simulink model "subsampling"  (R2025b)
settings: Solver=FixedStepAuto  StartTime=0.0  StopTime=9.999  RelTol=1e-3
model workspace (MAT data in the model file):
  Ts = 0.001
libraries: subsystems x1
settings Model: Creator=karadeli  LastModifiedBy=karadeli

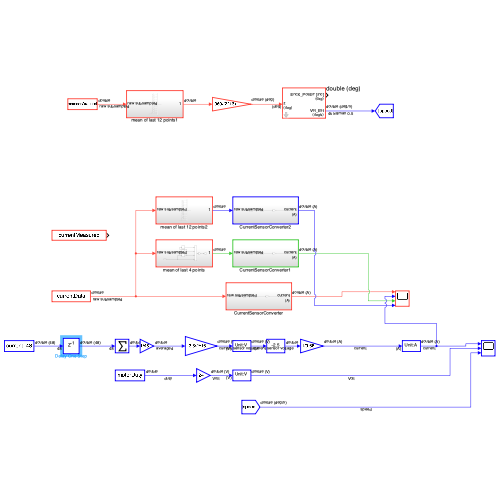
[thumbnail: Simulink's stored preview of the top-level diagram]
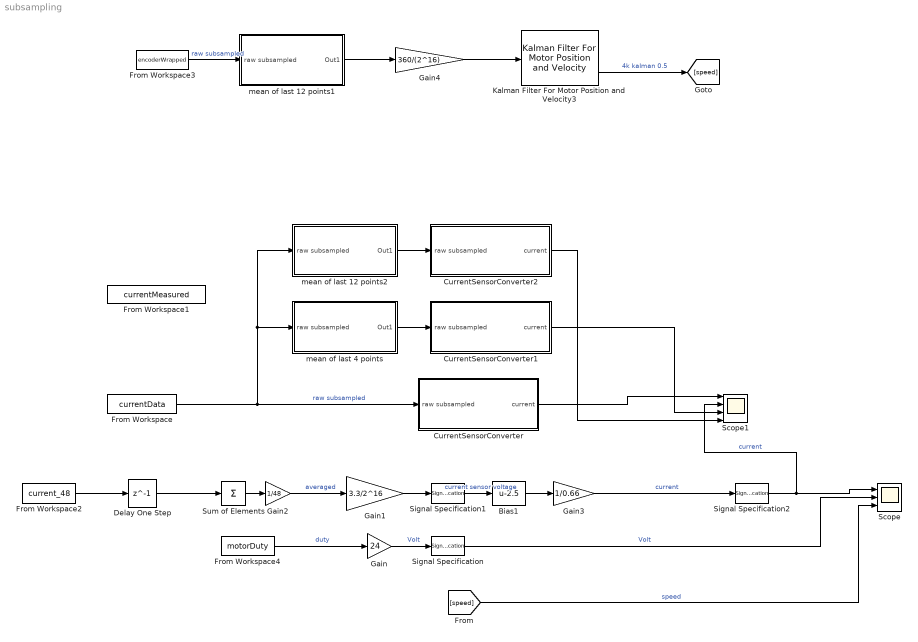
== system subsampling ==
  Bias1 : Bias  Bias=-2.5  SaturateOnIntegerOverflow=off
  CurrentSensorConverter : Subsystem
  CurrentSensorConverter1 : Subsystem
  CurrentSensorConverter2 : Subsystem
  Delay One Step : Delay  DelayLength=1  InitialCondition=2.5/3.3*2^16
  From Workspace : FromWorkspace  VariableName=currentData  SampleTime=1e-3/48  Interpolate=off  OutputAfterFinalValue=Holding final value
  From Workspace1 : FromWorkspace  VariableName=currentMeasured  SampleTime=1e-3/48  Interpolate=off  OutputAfterFinalValue=Holding final value
  From Workspace2 : FromWorkspace  VariableName=current_48  SampleTime=1e-3  Interpolate=off  OutputAfterFinalValue=Holding final value
  From Workspace3 : FromWorkspace  VariableName=encoderWrapped  SampleTime=1e-3/48  Interpolate=off  OutputAfterFinalValue=Holding final value
  From Workspace4 : FromWorkspace  VariableName=motorDuty  SampleTime=1e-3  Interpolate=off  OutputAfterFinalValue=Holding final value
  Gain : Gain  Gain=24
  Gain1 : Gain  Gain=3.3/2^16
  Gain2 : Gain  Gain=1/48
  Gain3 : Gain  Gain=1/0.66
  Gain4 : Gain  Gain=360/(2^16)
  Kalman Filter For Motor Position and Velocity3 : subsystems/Kalman Filter For Motor Position and Velocity  Ts=1e-3/4  lambda_RQ=0.5
  Scope : Scope  NumInputPorts=3
      settings: ActiveDisplayYMinimum=-2.2944343090057369  ActiveDisplayYMaximum=1.5207278728485107
  Scope1 : Scope  NumInputPorts=4
      settings: ActiveDisplayYMinimum=-0.17064403441405929  ActiveDisplayYMaximum=0.16131402448510473
  Signal Specification : SignalSpecification  Unit=V
  Signal Specification1 : SignalSpecification  Unit=V
  Signal Specification2 : SignalSpecification  Unit=A
  Sum of Elements : Sum  Inputs=+
  mean of last 12 points1 : Subsystem
  mean of last 12 points2 : Subsystem
  mean of last 4 points : Subsystem
  wires:
  Sum of Elements/1 -> Gain2/1
  From Workspace2/1 -> Delay One Step/1
  Kalman Filter For Motor Position and Velocity3/2 -> [speed]  "4k kalman 0.5"
  mean of last 12 points1/1(Out1) -> Gain4/1
  Gain4/1 -> Kalman Filter For Motor Position and Velocity3/1
  Gain2/1 -> Gain1/1  "averaged"
  Gain1/1 -> Signal Specification1/1
  Bias1/1 -> Gain3/1
  Gain3/1 -> Signal Specification2/1  "current"
  From Workspace4/1 -> Gain/1  "duty"
  From Workspace3/1 -> mean of last 12 points1/1(raw subsampled)  "raw subsampled"
  [speed] -> Scope/3  "speed"
  Gain/1 -> Signal Specification/1  "Volt"
  Signal Specification/1 -> Scope/2  "Volt"
  Signal Specification1/1 -> Bias1/1  "current sensor voltage"
  Signal Specification2/1 -> Scope1/2, Scope/1  "current"
  From Workspace/1 -> CurrentSensorConverter/1(raw subsampled), mean of last 12 points2/1(raw subsampled), mean of last 4 points/1(raw subsampled)  "raw subsampled"
  CurrentSensorConverter/1(current) -> Scope1/1
  mean of last 4 points/1(Out1) -> CurrentSensorConverter1/1(raw subsampled)
  CurrentSensorConverter1/1(current) -> Scope1/3
  mean of last 12 points2/1(Out1) -> CurrentSensorConverter2/1(raw subsampled)
  CurrentSensorConverter2/1(current) -> Scope1/4
  Delay One Step/1 -> Sum of Elements/1

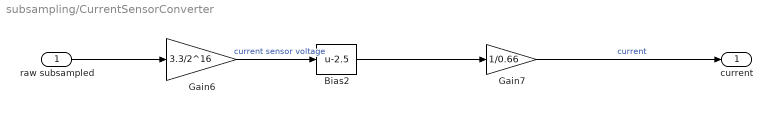
== system subsampling/CurrentSensorConverter ==
  raw subsampled : Inport
  Bias2 : Bias  Bias=-2.5  SaturateOnIntegerOverflow=off
  Gain6 : Gain  Gain=3.3/2^16
  Gain7 : Gain  Gain=1/0.66
  current : Outport  Unit=A
  wires:
  raw subsampled/1 -> Gain6/1
  Gain7/1 -> current/1  "current"
  Bias2/1 -> Gain7/1
  Gain6/1 -> Bias2/1  "current sensor voltage"

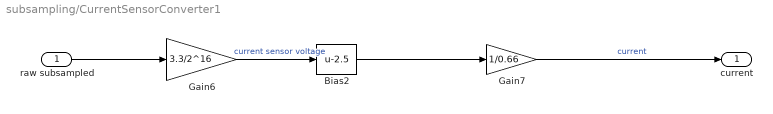
== system subsampling/CurrentSensorConverter1 ==
  raw subsampled : Inport
  Bias2 : Bias  Bias=-2.5  SaturateOnIntegerOverflow=off
  Gain6 : Gain  Gain=3.3/2^16
  Gain7 : Gain  Gain=1/0.66
  current : Outport  Unit=A
  wires:
  Gain6/1 -> Bias2/1  "current sensor voltage"
  Bias2/1 -> Gain7/1
  Gain7/1 -> current/1  "current"
  raw subsampled/1 -> Gain6/1

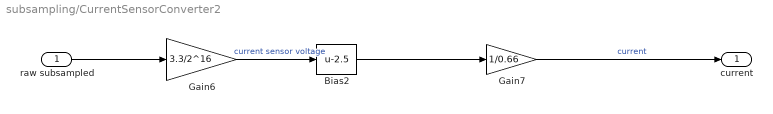
== system subsampling/CurrentSensorConverter2 ==
  raw subsampled : Inport
  Bias2 : Bias  Bias=-2.5  SaturateOnIntegerOverflow=off
  Gain6 : Gain  Gain=3.3/2^16
  Gain7 : Gain  Gain=1/0.66
  current : Outport  Unit=A
  wires:
  raw subsampled/1 -> Gain6/1
  Gain7/1 -> current/1  "current"
  Bias2/1 -> Gain7/1
  Gain6/1 -> Bias2/1  "current sensor voltage"

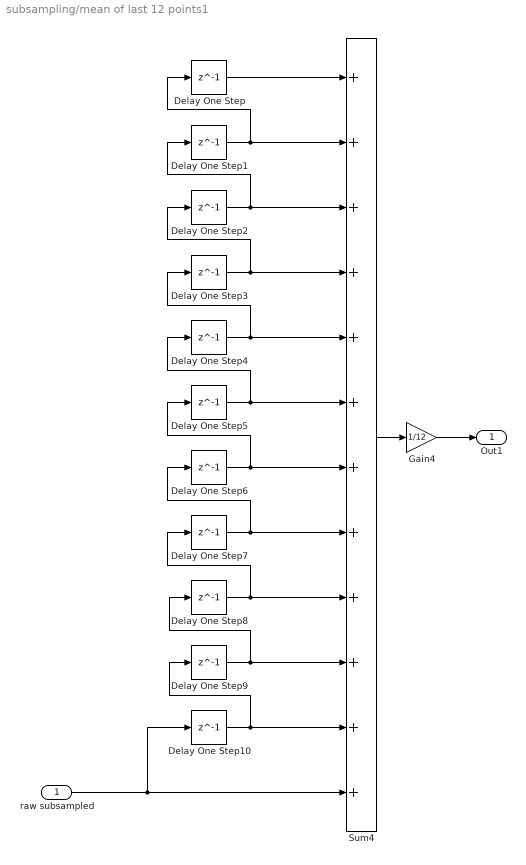
== system subsampling/mean of last 12 points1 ==
  raw subsampled : Inport
  Delay One Step{,1..10} (11 alike) : Delay  DelayLength=1
  Gain4 : Gain  Gain=1/12
  Sum4 : Sum  Inputs=12
  Out1 : Outport
  wires:
  Sum4/1 -> Gain4/1
  Gain4/1 -> Out1/1
  raw subsampled/1 -> Sum4/12, Delay One Step10/1
  Delay One Step8/1 -> Sum4/9, Delay One Step7/1
  Delay One Step7/1 -> Sum4/8, Delay One Step6/1
  Delay One Step6/1 -> Sum4/7, Delay One Step5/1
  Delay One Step5/1 -> Sum4/6, Delay One Step4/1
  Delay One Step4/1 -> Sum4/5, Delay One Step3/1
  Delay One Step3/1 -> Sum4/4, Delay One Step2/1
  Delay One Step2/1 -> Sum4/3, Delay One Step1/1
  Delay One Step1/1 -> Sum4/2, Delay One Step/1
  Delay One Step/1 -> Sum4/1
  Delay One Step9/1 -> Sum4/10, Delay One Step8/1
  Delay One Step10/1 -> Sum4/11, Delay One Step9/1

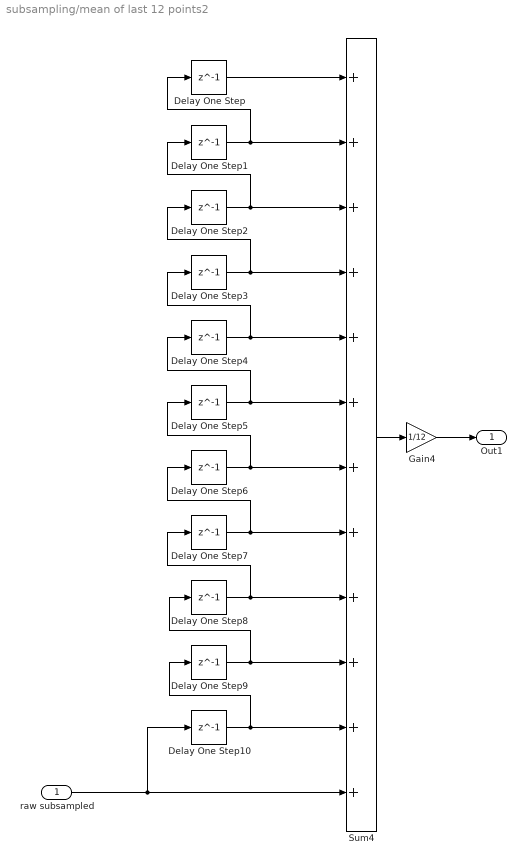
== system subsampling/mean of last 12 points2 ==
  raw subsampled : Inport
  Delay One Step{,1..10} (11 alike) : Delay  DelayLength=1
  Gain4 : Gain  Gain=1/12
  Sum4 : Sum  Inputs=12
  Out1 : Outport  SampleTime=1e-3/4
  wires:
  Delay One Step10/1 -> Delay One Step9/1, Sum4/11
  Delay One Step9/1 -> Delay One Step8/1, Sum4/10
  Delay One Step/1 -> Sum4/1
  Delay One Step1/1 -> Delay One Step/1, Sum4/2
  Delay One Step2/1 -> Delay One Step1/1, Sum4/3
  Delay One Step3/1 -> Delay One Step2/1, Sum4/4
  Delay One Step4/1 -> Delay One Step3/1, Sum4/5
  Delay One Step5/1 -> Delay One Step4/1, Sum4/6
  Delay One Step6/1 -> Delay One Step5/1, Sum4/7
  Delay One Step7/1 -> Delay One Step6/1, Sum4/8
  Delay One Step8/1 -> Delay One Step7/1, Sum4/9
  raw subsampled/1 -> Delay One Step10/1, Sum4/12
  Gain4/1 -> Out1/1
  Sum4/1 -> Gain4/1

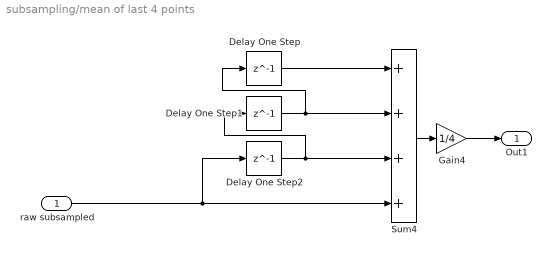
== system subsampling/mean of last 4 points ==
  raw subsampled : Inport  SampleTime=1e-3/48
  Delay One Step : Delay  DelayLength=1
  Delay One Step1 : Delay  DelayLength=1
  Delay One Step2 : Delay  DelayLength=1
  Gain4 : Gain  Gain=1/4
  Sum4 : Sum  Inputs=++++
  Out1 : Outport  SampleTime=1e-3/12
  wires:
  Gain4/1 -> Out1/1
  Delay One Step/1 -> Sum4/1
  Sum4/1 -> Gain4/1
  Delay One Step1/1 -> Delay One Step/1, Sum4/2
  raw subsampled/1 -> Delay One Step2/1, Sum4/4
  Delay One Step2/1 -> Delay One Step1/1, Sum4/3
